simulink model "fahdl"  (R2015a)
settings: Solver=ode45  StartTime=0.0  StopTime=10.0  RelTol=1e-3
settings Model: Creator=Shravankumar  LastModifiedBy=Shravankumar

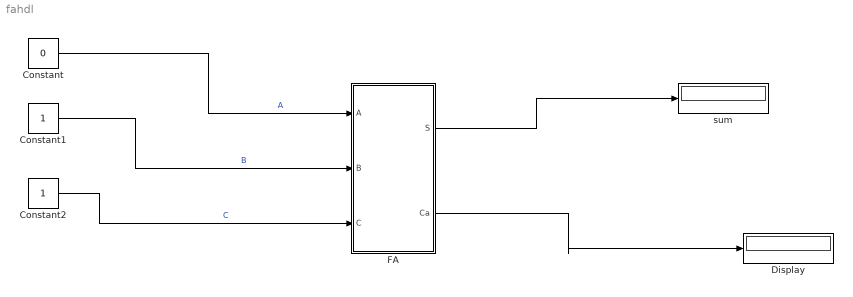
== system fahdl ==
  Constant : Constant  Value=0
  Constant1 : Constant
  Constant2 : Constant
  Display : Display
  FA : Subsystem
  sum : Display
  wires:
  Constant/1 -> FA/1(A)  "A"
  Constant1/1 -> FA/2(B)  "B"
  Constant2/1 -> FA/3(C)  "C"
  FA/1(S) -> sum/1
  FA/2(Ca) -> Display/1

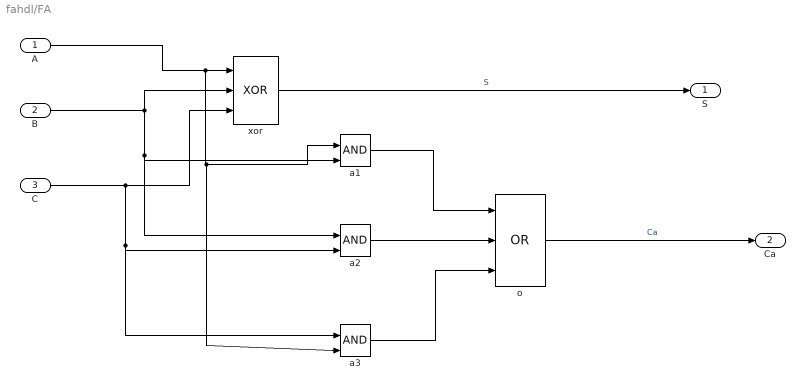
== system fahdl/FA ==
  A : Inport
  B : Inport  Port=2
  C : Inport  Port=3
  a1 : Logic  IconShape=distinctive  AllPortsSameDT=off  OutDataTypeStr=boolean
  a2 : Logic  IconShape=distinctive  AllPortsSameDT=off  OutDataTypeStr=boolean
  a3 : Logic  IconShape=distinctive  AllPortsSameDT=off  OutDataTypeStr=boolean
  o : Logic  Operator=OR  Inputs=3  IconShape=distinctive  AllPortsSameDT=off  OutDataTypeStr=boolean
  xor : Logic  Operator=XOR  Inputs=3  IconShape=distinctive  AllPortsSameDT=off  OutDataTypeStr=boolean
  S : Outport
  Ca : Outport  Port=2
  wires:
  A/1 -> a3/2, a1/1, xor/1
  C/1 -> a3/1, a2/2, xor/3
  xor/1 -> S/1  "S"
  o/1 -> Ca/1  "Ca"
  a2/1 -> o/2
  a3/1 -> o/3
  B/1 -> xor/2, a2/1, a1/2
  a1/1 -> o/1
